simulink model "circle_edit_g"  (R2020b)
settings: Solver=ode5  StartTime=0.0  StopTime=30  FixedStep=0.1  RelTol=1e-3
settings Model: Creator=skets  LastModifiedBy=skets
settings SolverCC: ConcurrentTasks=on  PositivePriorityOrder=on
settings DataIOCC: ReturnWorkspaceOutputs=off
settings OptimizationCC: DefaultParameterBehavior=Inlined  UseDivisionForNetSlopeComputation=on  GainParamInheritBuiltInType=on  UseFloatMulNetSlope=on  InlineInvariantSignals=on  PassReuseOutputArgsAs=Individual arguments  ZeroExternalMemoryAtStartup=off  ZeroInternalMemoryAtStartup=off  NoFixptDivByZeroProtection=on  EfficientFloat2IntCast=on  LifeSpan=1  OptimizeBlockOrder=speed  DifferentSizesBufferReuse=on  EfficientTunableParamExpr=on
settings DebuggingCC: ParameterTunabilityLossMsg=error  ArithmeticOperatorsInVariantConditions=warning
settings HardwareCC: ProdBitPerPointer=32  ProdBitPerSizeT=32  ProdBitPerPtrDiffT=32  ProdLargestAtomicInteger=Long  ProdLargestAtomicFloat=Double  ProdWordSize=32  ProdLongLongMode=on  ProdHWDeviceType=ARM Compatible->ARM Cortex-M
settings SFSimCC: SimUseLocalCustomCode=off  MATLABDynamicMemAlloc=off  CustomCodeUndefinedFunction=UseInterfaceOnly
settings RTWCC: Description=Embedded Coder  SystemTargetFile=ert.tlc  PackageName=dynamic_circle  TemplateMakefile=ert_default_tmf  RTWUseLocalCustomCode=off  Toolchain=GNU Tools for ARM Embedded Processors  BuildConfiguration=Debug
settings CodeAppCC: ForceParamTrailComments=on  IgnoreCustomStorageClasses=off  OperatorAnnotations=on  SimulinkDataObjDesc=on  SFDataObjDesc=on  CustomSymbolStrGlobalVar=rt$N$M  CustomSymbolStrType=$N$M  CustomSymbolStrFcn=$N$M$F  CustomSymbolStrMacro=$N$M  InsertBlockDesc=on
settings ERTTargetCC: TargetLangStandard=C99 (ISO)  GenerateSampleERTMain=on  IncludeMdlTerminateFcn=off  CombineSignalStateStructs=on  SupportComplex=off  SupportContinuousTime=on  SupportNonInlinedSFcns=on  InlinedParameterPlacement=NonHierarchical  TargetOS=NativeThreadsExample  ERTCustomFileTemplate=example_file_process.tlc  ERTFilePackagingFormat=CompactWithDataFile

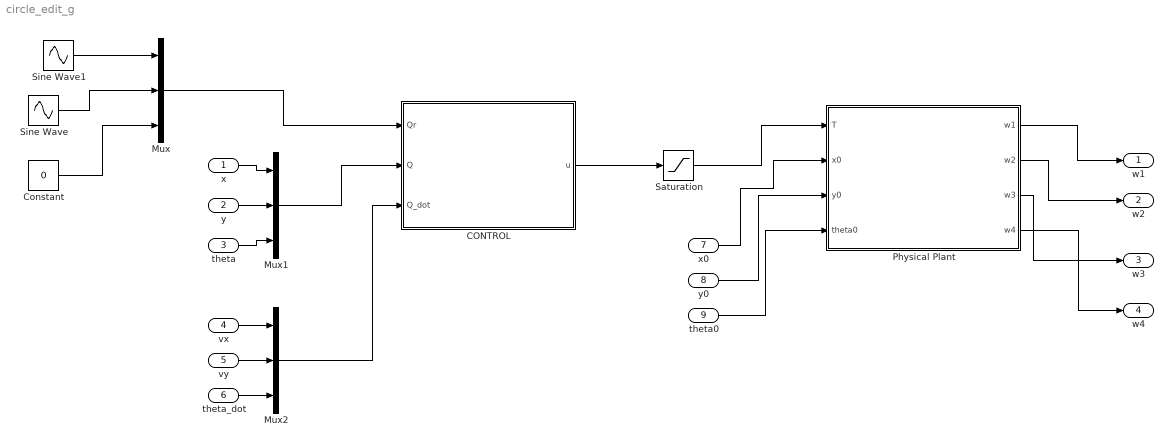
== system circle_edit_g ==
  x : Inport
  y : Inport  Port=2
  theta : Inport  Port=3
  vx : Inport  Port=4
  vy : Inport  Port=5
  theta_dot : Inport  Port=6
  x0 : Inport  Port=7
  y0 : Inport  Port=8
  theta0 : Inport  Port=9
  CONTROL : Subsystem
  Constant : Constant  Value=0
  Mux : Mux  Inputs=3
  Mux1 : Mux  Inputs=3
  Mux2 : Mux  Inputs=3
  Physical Plant : Subsystem
  Saturation : Saturate  UpperLimit=5  LowerLimit=-5
  Sine Wave : Sin  Amplitude=0.25  Bias=0.6  Frequency=2*pi/30
  Sine Wave1 : Sin  Amplitude=-0.25  Bias=1.5  Frequency=2*pi/30  Phase=pi/2
  w1 : Outport  VectorParamsAs1DForOutWhenUnconnected=off
  w2 : Outport  Port=2  VectorParamsAs1DForOutWhenUnconnected=off
  w3 : Outport  Port=3  VectorParamsAs1DForOutWhenUnconnected=off
  w4 : Outport  Port=4  VectorParamsAs1DForOutWhenUnconnected=off
  wires:
  Sine Wave/1 -> Mux/2
  Constant/1 -> Mux/3
  Sine Wave1/1 -> Mux/1
  Mux/1 -> CONTROL/1(Qr)
  CONTROL/1(u) -> Saturation/1
  Saturation/1 -> Physical Plant/1(T)
  Physical Plant/1(w1) -> w1/1
  Physical Plant/2(w2) -> w2/1
  Physical Plant/3(w3) -> w3/1
  Physical Plant/4(w4) -> w4/1
  x/1 -> Mux1/1
  y/1 -> Mux1/2
  Mux1/1 -> CONTROL/2(Q)
  Mux2/1 -> CONTROL/3(Q_dot)
  vx/1 -> Mux2/1
  theta_dot/1 -> Mux2/3
  vy/1 -> Mux2/2
  theta/1 -> Mux1/3
  x0/1 -> Physical Plant/2(x0)
  y0/1 -> Physical Plant/3(y0)
  theta0/1 -> Physical Plant/4(theta0)

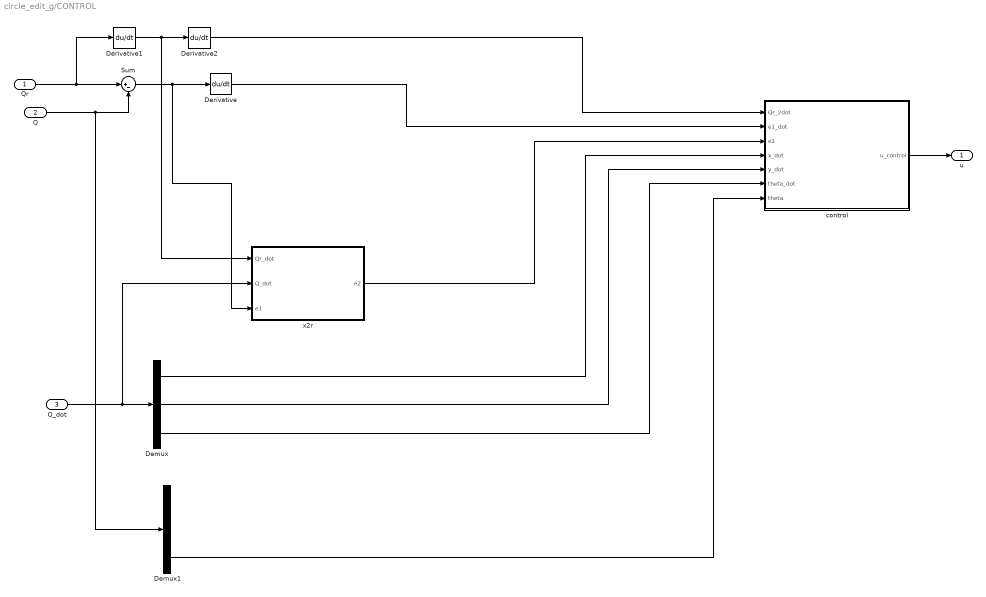
== system circle_edit_g/CONTROL ==
  Qr : Inport
  Q : Inport  Port=2  PortDimensions=3
  Q_dot : Inport  Port=3
  Demux : Demux  Outputs=3
  Demux1 : Demux  Outputs=3
  Derivative : Derivative
  Derivative1 : Derivative
  Derivative2 : Derivative
  Sum : Sum  Inputs=|+-
  control : MATLAB Function  TreatAsAtomicUnit=on
  x2r : MATLAB Function  TreatAsAtomicUnit=on
  u : Outport  VectorParamsAs1DForOutWhenUnconnected=off
  wires:
  Qr/1 -> Derivative1/1, Sum/1
  Derivative1/1 -> x2r/1(Qr_dot), Derivative2/1
  control/1(u_control) -> u/1
  Q/1 -> Demux1/1, Sum/2
  Q_dot/1 -> x2r/2(Q_dot), Demux/1
  Demux/1 -> control/4(x_dot)
  Demux/2 -> control/5(y_dot)
  Demux/3 -> control/6(theta_dot)
  Demux1/3 -> control/7(theta)
  Sum/1 -> x2r/3(e1), Derivative/1
  Derivative2/1 -> control/1(Qr_2dot)
  Derivative/1 -> control/2(e1_dot)
  x2r/1(e2) -> control/3(e2)

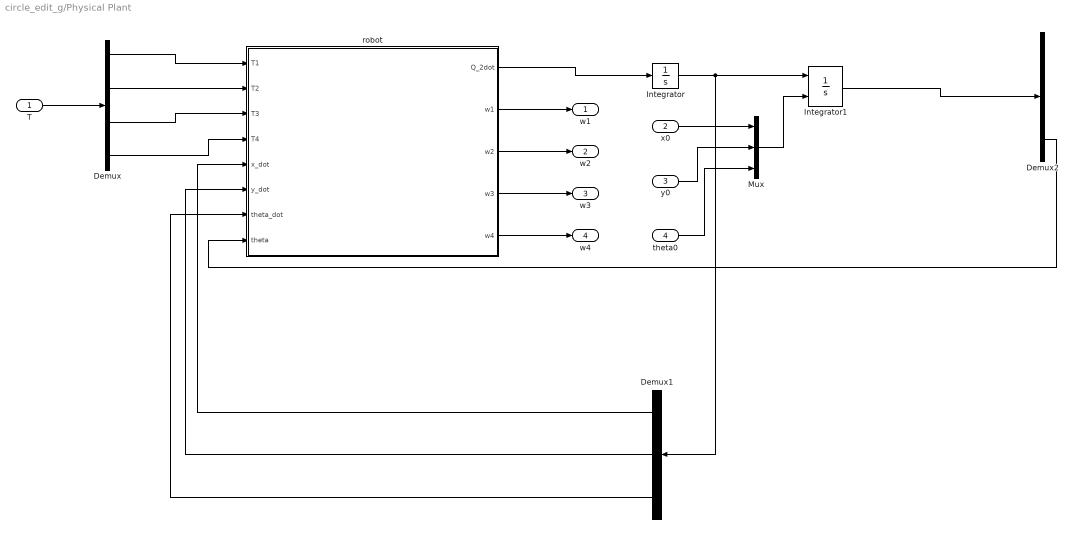
== system circle_edit_g/Physical Plant ==
  T : Inport  PortDimensions=4
  x0 : Inport  Port=2  PortDimensions=1
  y0 : Inport  Port=3  PortDimensions=1
  theta0 : Inport  Port=4  PortDimensions=1
  Demux : Demux
  Demux1 : Demux  Outputs=3
  Demux2 : Demux  Outputs=3
  Integrator : Integrator
  Integrator1 : Integrator  InitialConditionSource=external  InitialCondition=[0.5 1 0]
  Mux : Mux  Inputs=3
  robot : MATLAB Function  TreatAsAtomicUnit=on
  w1 : Outport  VectorParamsAs1DForOutWhenUnconnected=off
  w2 : Outport  Port=2  VectorParamsAs1DForOutWhenUnconnected=off
  w3 : Outport  Port=3  VectorParamsAs1DForOutWhenUnconnected=off
  w4 : Outport  Port=4  VectorParamsAs1DForOutWhenUnconnected=off
  wires:
  Demux/1 -> robot/1(T1)
  Demux/2 -> robot/2(T2)
  Demux/3 -> robot/3(T3)
  Demux/4 -> robot/4(T4)
  robot/1(Q_2dot) -> Integrator/1
  Integrator/1 -> Demux1/1, Integrator1/1
  Demux1/1 -> robot/5(x_dot)
  Demux1/2 -> robot/6(y_dot)
  Demux1/3 -> robot/7(theta_dot)
  Integrator1/1 -> Demux2/1
  Demux2/3 -> robot/8(theta)
  T/1 -> Demux/1
  robot/2(w1) -> w1/1
  robot/3(w2) -> w2/1
  robot/4(w3) -> w3/1
  robot/5(w4) -> w4/1
  Mux/1 -> Integrator1/2
  x0/1 -> Mux/1
  y0/1 -> Mux/2
  theta0/1 -> Mux/3

== matlab function circle_edit_g/Physical Plant/robot ==
  data: T1 input; Q_2dot output; T2 input; T3 input; T4 input; x_dot input; y_dot input; theta_dot input; theta input; w1 output; w2 output; w3 output; w4 output
function [Q_2dot,w1,w2,w3,w4]  = fcn(T1, T2, T3, T4,x_dot,y_dot,theta_dot,theta)

m=5;
I=5;
Ib=0.1;
l1= 0.3;
l2=0.3;
r=0.048;
g=9.8;
u=0.01;
N = m*g/4;
M=[(m+4*Ib/(r*r)) 0 0; 0 (m+4*Ib/(r*r)) 0; 0 0 (I+4*Ib*(l1+l2)*(l1+l2)/(r*r))];
C= [(m+4*Ib/(r*r))*y_dot*theta_dot;-(m+4*Ib/(r*r))*x_dot*theta_dot;0 ];
B=(1/r)*[(cos(theta)+sin(theta)) (cos(theta)-sin(theta)) (cos(theta)+sin(theta)) (cos(theta)-sin(theta));
         (-cos(theta)+sin(theta)) (cos(theta)+sin(theta)) (-cos(theta)+sin(theta)) (cos(theta)+sin(theta)); 
         (-(l1+l2)) (l1+l2) (l1+l2) (-(l1+l2)) ];
T=[T1;T2;T3;T4];
xm= cos(theta)*x_dot+sin(theta)*y_dot;
ym= -sin(theta)*x_dot+cos(theta)*y_dot;
w1 = (1/r)*(xm-ym-(l1+l2)*theta_dot);
w2 = (1/r)*(xm+ym+(l1+l2)*theta_dot);
w3 = (1/r)*(xm-ym+(l1+l2)*theta_dot);
w4 = (1/r)*(xm+ym-(l1+l2)*theta_dot);
w_max = 2.304;
if w1 > w_max
    w1 = w_max; %w = 20.83
elseif w1 < -w_max
    w1 = -w_max;
end
if w2 > w_max
    w2 = w_max;
elseif w2 < -w_max
    w2 = -w_max;
end
if w3 > w_max
    w3 = w_max;
elseif w3 < -w_max
    w3 = -w_max;
end
if w4 > w_max
    w4 = w_max;
elseif w4 < -w_max
    w4 = -w_max;
end
Xi=[u*r*N*sign(w1);u*r*N*sign(w2);u*r*N*sign(w3);u*N*r*sign(w4)];

Q_2dot=inv(M)*(B*T-C-B*Xi);

== matlab function circle_edit_g/CONTROL/control ==
  data: Qr_2dot input; u_control output; e1_dot input; e2 input; x_dot input; y_dot input; theta_dot input; theta input
function u_control = fcn(Qr_2dot,e1_dot,e2,x_dot,y_dot,theta_dot,theta)

m=5;
I=5;
Ib=0.1;
l1= 0.3;
l2=0.3;
r=0.048;
g=9.8;
u=0.01;
N = m*g/4;
M=[(m+4*Ib/(r*r)) 0 0; 0 (m+4*Ib/(r*r)) 0; 0 0 (I+4*Ib*(l1+l2)*(l1+l2)/(r*r))];
C= [(m+4*Ib/(r*r))*y_dot*theta_dot;-(m+4*Ib/(r*r))*x_dot*theta_dot;0 ];
B=(1/r)*[(cos(theta)+sin(theta)) (cos(theta)-sin(theta)) (cos(theta)+sin(theta)) (cos(theta)-sin(theta));
    (-cos(theta)+sin(theta)) (cos(theta)+sin(theta)) (-cos(theta)+sin(theta)) (cos(theta)+sin(theta)); 
    (-(l1+l2)) (l1+l2) (l1+l2) (-(l1+l2)) ];

xm= cos(theta)*x_dot+sin(theta)*y_dot;
ym= -sin(theta)*x_dot+cos(theta)*y_dot;
w1 = (1/r)*(xm-ym-(l1+l2)*theta_dot);
w2 = (1/r)*(xm+ym+(l1+l2)*theta_dot);
w3 = (1/r)*(xm-ym+(l1+l2)*theta_dot);
w4 = (1/r)*(xm+ym-(l1+l2)*theta_dot);
w_max = 2.304;
if w1 > w_max
    w1 = w_max; %w = 20.83
elseif w1 < -w_max
    w1 = -w_max;
end
if w2 > w_max
    w2 = w_max;
elseif w2 < -w_max
    w2 = -w_max;
end
if w3 > w_max
    w3 = w_max;
elseif w3 < -w_max
    w3 = -w_max;
end
if w4 > w_max
    w4 = w_max;
elseif w4 < -w_max
    w4 = -w_max;
end
Xi=[u*r*N*sign(w1);u*r*N*sign(w2);u*r*N*sign(w3);u*N*r*sign(w4)];

k1 = [4 0 0;
      0 4 0;
      0 0 4];
k2 = [4 0 0;
      0 4 0;
      0 0 4];
  
u_control = B'*inv(B*B')*M*((Qr_2dot+k1*e1_dot)+inv(M)*C+inv(M)*B*Xi+k2*e2);

== matlab function circle_edit_g/CONTROL/x2r ==
  data: Qr_dot input; Q_dot input; e2 output; e1 input
function e2  = fcn(Qr_dot,Q_dot,e1)

k1 = [4 0 0;
      0 4 0;
      0 0 4];
 
%x2r_dot = (Qr_2dot+k1*e1_dot);
x2r = Qr_dot + k1*e1;
e2 = x2r - Q_dot;
